simulink model "targeting_speed_angles"  (R2020a)
settings: Solver=VariableStepAuto  StartTime=0.0  StopTime=10.0  RelTol=1e-3
settings Model: Creator=Tamer  LastModifiedBy=Tamer
settings SolverCC: ZeroCrossControl=DisableAll
settings DataIOCC: SaveOutput=off  SaveTime=off
settings GRTTargetCC: CombineOutputUpdateFcns=off  MatFileLogging=off

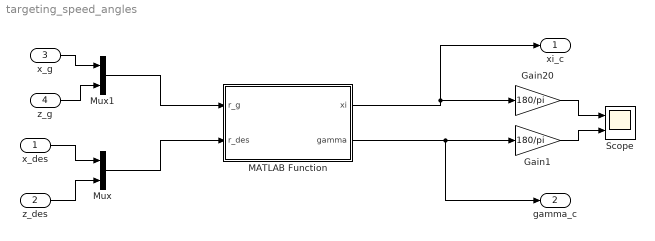
== system targeting_speed_angles ==
  x_des : Inport
  z_des : Inport  Port=2
  x_g : Inport  Port=3
  z_g : Inport  Port=4
  Gain1 : Gain  Gain=180/pi
  Gain20 : Gain  Gain=180/pi
  MATLAB Function : MATLAB Function  TreatAsAtomicUnit=on
  Mux : Mux  Inputs=3
  Mux1 : Mux  Inputs=3
  Scope : Scope  NumInputPorts=2
  xi_c : Outport
  gamma_c : Outport  Port=2
  wires:
  x_des/1 -> Mux/1
  z_des/1 -> Mux/3
  x_g/1 -> Mux1/1
  z_g/1 -> Mux1/3
  Mux1/1 -> MATLAB Function/1(r_g)
  Mux/1 -> MATLAB Function/2(r_des)
  MATLAB Function/2(gamma) -> gamma_c/1, Gain1/1
  MATLAB Function/1(xi) -> Gain20/1, xi_c/1
  Gain20/1 -> Scope/1
  Gain1/1 -> Scope/2

== matlab function targeting_speed_angles/MATLAB Function ==
  data: r_g input; xi output; r_des input; gamma output
function [xi, gamma] = fcn(r_g, r_des)
delta_r = r_des - r_g;
xi = atan2(-delta_r(3), delta_r(1));
gamma = 0;
